simulink model "sampleModel2021"  (R2023a)
settings: Solver=VariableStepAuto  StartTime=0.0  StopTime=10.0  RelTol=1e-3
libraries: hdlsllib x4
settings Model: Creator=user1  LastModifiedBy=user1

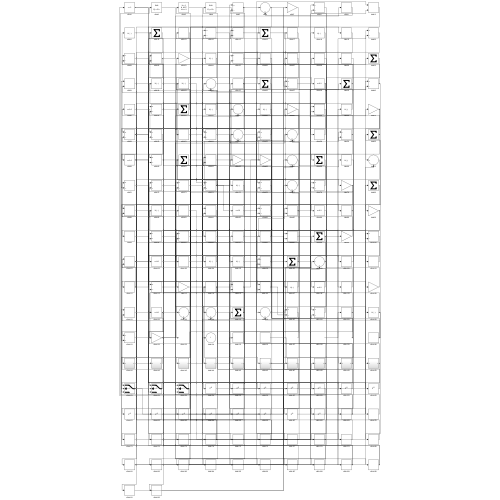
[thumbnail: Simulink's stored preview of the top-level diagram]
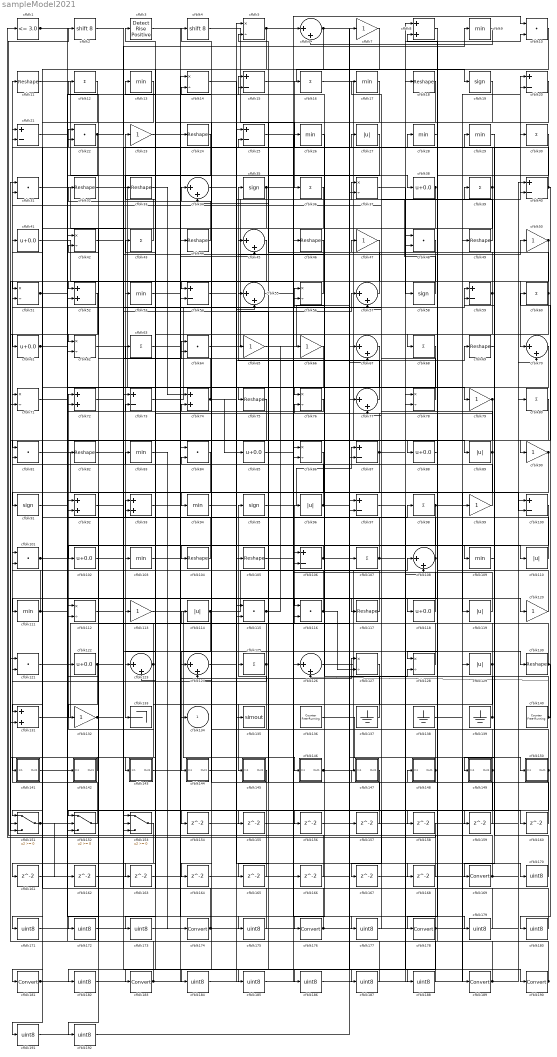
== system sampleModel2021 ==
  cfblk1 : hdlsllib/Logic and Bit Operations/Compare To Constant  relop=<=  const=3.0  OutDataTypeStr=boolean
  cfblk{10,22,31,48,64,81,84,101,115..116,121} (11 alike) : DotProduct  OutDataTypeStr=Inherit: Inherit via internal rule
  cfblk{15,20..21,25,40,54,59,73,87,97,100,106} (12 alike) : Sum  Inputs=+-
  cfblk{38,41,61,85,88,102,118,122} (8 alike) : Bias  Bias=0.0  SaturateOnIntegerOverflow=off
  cfblk{9,13,17,26,28..29,53,83,94,103,109,111} (12 alike) : MinMax
  cfblk{11,18,24,32..33,44,46,49,69,75,82,104..105,117,130} (15 alike) : Reshape
  cfblk{12,16,30,36,39,43,60,63,68,80,98,107,125} (13 alike) : Sum  Inputs=+
  cfblk{6,34,45,55,57,67,70,77,108,123..124,126} (12 alike) : Sum  Inputs=|++
  cfblk{27,89,96,110,114,119,129} (7 alike) : Abs  SaturateOnIntegerOverflow=off
  cfblk{5,14,37,42,51,56,62,71,76,78,86,112,127..128} (14 alike) : Product  Inputs=*/  RndMeth=Zero  SaturateOnIntegerOverflow=on
  cfblk{7,23,47,50,65..66,79,90,99,113,120,132} (12 alike) : Gain
  cfblk{8,52,72,74,92..93,131} (7 alike) : Sum
  cfblk133 : Terminator
  cfblk135 : ToWorkspace  VariableName=simout  SaveFormat=Timeseries  SampleTime=-1
  cfblk136 : hdlsllib/Sources/Counter Free-Running  NumBits=16  tsamp=-1
  cfblk137 : Ground
  cfblk138 : Ground
  cfblk139 : Ground
  cfblk140 : hdlsllib/Sources/Counter Free-Running  NumBits=16  tsamp=-1
  cfblk141 : Subsystem
      settings: LibrarySourceBlock=|
      | hdlsllib/Ports &
      | Subsystems/Subsystem
  cfblk142 : Subsystem
      settings: LibrarySourceBlock=|
      | hdlsllib/Ports &
      | Subsystems/Subsystem
  cfblk143 : Subsystem
      settings: LibrarySourceBlock=|
      | hdlsllib/Ports &
      | Subsystems/Subsystem
  cfblk144 : Subsystem
      settings: LibrarySourceBlock=|
      | hdlsllib/Ports &
      | Subsystems/Subsystem
  cfblk145 : Subsystem
      settings: LibrarySourceBlock=|
      | hdlsllib/Ports &
      | Subsystems/Subsystem
  cfblk146 : Subsystem
      settings: LibrarySourceBlock=|
      | hdlsllib/Ports &
      | Subsystems/Subsystem
  cfblk147 : Subsystem
      settings: LibrarySourceBlock=|
      | hdlsllib/Ports &
      | Subsystems/Subsystem
  cfblk148 : Subsystem
      settings: LibrarySourceBlock=|
      | hdlsllib/Ports &
      | Subsystems/Subsystem
  cfblk149 : Subsystem
      settings: LibrarySourceBlock=|
      | hdlsllib/Ports &
      | Subsystems/Subsystem
  cfblk150 : Subsystem
      settings: LibrarySourceBlock=|
      | hdlsllib/Ports &
      | Subsystems/Subsystem
  cfblk151 : Switch  SaturateOnIntegerOverflow=off  InputSameDT=off
  cfblk152 : Switch  SaturateOnIntegerOverflow=off  InputSameDT=off
  cfblk153 : Switch  SaturateOnIntegerOverflow=off  InputSameDT=off
  cfblk{154..168} (15 alike) : Delay  SampleTime=1
  cfblk{169,174,176,178,181,183,189..190} (8 alike) : DataTypeConversion  SaturateOnIntegerOverflow=off  RndMeth=Floor
  cfblk{170..173,175,177,179..180,182,184..188,191..192} (16 alike) : DataTypeConversion  OutDataTypeStr=uint8  SaturateOnIntegerOverflow=off  RndMeth=Floor
  cfblk{19,35,58,91,95} (5 alike) : Signum
  cfblk2 : ArithShift  BitShiftNumber=8
  cfblk3 : hdlsllib/Logic and Bit Operations/Detect Rise Positive  vinit=0  OutDataTypeStr=boolean
  cfblk4 : ArithShift  BitShiftNumber=8
  cfblk134 : Outport  VectorParamsAs1DForOutWhenUnconnected=off
  wires:
  cfblk73/1 -> cfblk56/1
  cfblk152/1 -> cfblk11/1
  cfblk70/1 -> cfblk104/1
  cfblk11/1 -> cfblk38/1
  cfblk24/1 -> cfblk133/1
  cfblk127/1 -> cfblk72/1
  cfblk77/1 -> cfblk35/1
  cfblk33/1 -> cfblk74/1
  cfblk56/1 -> cfblk51/1
  cfblk150/1(Out1) -> cfblk34/1, cfblk167/1
  cfblk90/1 -> cfblk124/2, cfblk172/1
  cfblk15/1 -> cfblk19/1
  cfblk59/1 -> cfblk94/1, cfblk34/2
  cfblk58/1 -> cfblk20/1
  cfblk26/1 -> cfblk76/1
  cfblk84/1 -> cfblk113/1
  cfblk69/1 -> cfblk149/1(In1)
  cfblk35/1 -> cfblk117/1, cfblk173/1
  cfblk97/1 -> cfblk190/1
  cfblk46/1 -> cfblk52/1
  cfblk16/1 -> cfblk89/1
  cfblk21/1 -> cfblk112/1
  cfblk64/1 -> cfblk37/1
  cfblk116/1 -> cfblk21/1, cfblk127/2
  cfblk121/1 -> cfblk24/1
  cfblk146/1(Out1) -> cfblk108/1, cfblk128/2
  cfblk145/1(Out1) -> cfblk2/1
  cfblk17/1 -> cfblk37/2
  cfblk95/1 -> cfblk87/1
  cfblk138/1 -> cfblk49/1
  cfblk129/1 -> cfblk145/1(In1), cfblk84/2
  cfblk131/1 -> cfblk7/1
  cfblk114/1 -> cfblk144/1(In1), cfblk18/1
  cfblk80/1 -> cfblk181/1
  cfblk19/1 -> cfblk75/1
  cfblk38/1 -> cfblk62/1, cfblk184/1
  cfblk79/1 -> cfblk76/2, cfblk151/3
  cfblk22/1 -> cfblk52/2, cfblk9/1
  cfblk68/1 -> cfblk123/1
  cfblk32/1 -> cfblk107/1
  cfblk43/1 -> cfblk23/1
  cfblk136/1 -> cfblk189/1
  cfblk47/1 -> cfblk176/1
  cfblk89/1 -> cfblk132/1, cfblk31/2
  cfblk130/1 -> cfblk96/1, cfblk180/1
  cfblk148/1(Out1) -> cfblk147/1(In1), cfblk125/1
  cfblk98/1 -> cfblk20/2, cfblk164/1
  cfblk10/1 -> cfblk123/2
  cfblk85/1 -> cfblk46/1
  cfblk109/1 -> cfblk59/1
  cfblk67/1 -> cfblk183/1
  cfblk30/1 -> cfblk118/1
  cfblk76/1 -> cfblk72/2
  cfblk86/1 -> cfblk91/1
  cfblk6/1 -> cfblk131/1, cfblk100/2
  cfblk78/1 -> cfblk51/2
  cfblk41/1 -> cfblk126/1
  cfblk101/1 -> cfblk15/2, cfblk175/1
  cfblk31/1 -> cfblk53/1
  cfblk82/1 -> cfblk50/1
  cfblk106/1 -> cfblk150/1(In1), cfblk102/1
  cfblk122/1 -> cfblk59/2, cfblk152/3
  cfblk126/1 -> cfblk78/1
  cfblk113/1 -> cfblk146/1(In1)
  cfblk99/1 -> cfblk71/1
  cfblk23/1 -> cfblk130/1
  cfblk40/1 -> cfblk16/1, cfblk90/1
  cfblk34/1 -> cfblk30/1
  cfblk71/1 -> cfblk120/1
  cfblk29/1 -> cfblk169/1
  cfblk44/1 -> cfblk32/1
  cfblk149/1(Out1) -> cfblk95/1, cfblk27/1, cfblk182/1
  cfblk110/1 -> cfblk43/1
  cfblk142/1(Out1) -> cfblk141/1(In1)
  cfblk103/1 -> cfblk44/1
  cfblk20/1 -> cfblk54/1
  cfblk1/1 -> cfblk109/1, cfblk79/1
  cfblk45/1 -> cfblk71/2
  cfblk105/1 -> cfblk6/1
  cfblk120/1 -> cfblk21/2
  cfblk91/1 -> cfblk142/1(In1)
  cfblk144/1(Out1) -> cfblk25/1
  cfblk52/1 -> cfblk131/2
  cfblk119/1 -> cfblk106/1
  cfblk137/1 -> cfblk45/1
  cfblk151/1 -> cfblk152/2, cfblk162/1
  cfblk93/1 -> cfblk45/2
  cfblk72/1 -> cfblk153/1
  cfblk4/1 -> cfblk36/1
  cfblk36/1 -> cfblk81/1
  cfblk117/1 -> cfblk33/1
  cfblk8/1 -> cfblk178/1
  cfblk5/1 -> cfblk92/2, cfblk10/1
  cfblk96/1 -> cfblk65/1, cfblk64/2, cfblk168/1
  cfblk60/1 -> cfblk28/1, cfblk143/1(In1)
  cfblk57/1 -> cfblk5/2
  cfblk143/1(Out1) -> cfblk127/1
  cfblk128/1 -> cfblk114/1
  cfblk108/1 -> cfblk13/1, cfblk151/1
  cfblk14/1 -> cfblk55/2
  cfblk66/1 -> cfblk111/1
  cfblk125/1 -> cfblk121/2, cfblk22/1, cfblk93/1
  cfblk100/1 -> cfblk112/2
  cfblk139/1 -> cfblk15/1, cfblk63/1
  cfblk107/1 -> cfblk110/1, cfblk26/1
  cfblk12/1 -> cfblk61/1
  cfblk140/1 -> cfblk56/2, cfblk126/2, cfblk60/1
  cfblk132/1 -> cfblk57/1, cfblk25/2
  cfblk81/1 -> cfblk119/1
  cfblk112/1 -> cfblk98/1
  cfblk74/1 -> cfblk69/1, cfblk22/2, cfblk116/2, cfblk85/1
  cfblk123/1 -> cfblk12/1, cfblk151/2
  cfblk61/1 -> cfblk153/3, cfblk160/1
  cfblk115/1 -> cfblk66/1, cfblk155/1
  cfblk39/1 -> cfblk4/1, cfblk116/1
  cfblk50/1 -> cfblk54/2, cfblk70/1
  cfblk18/1 -> cfblk103/1
  cfblk28/1 -> cfblk68/1
  cfblk51/1 -> cfblk86/2, cfblk115/2
  cfblk37/1 -> cfblk58/1
  cfblk94/1 -> cfblk40/2
  cfblk87/1 -> cfblk3/1, cfblk10/2, cfblk185/1
  cfblk62/1 -> cfblk105/1
  cfblk88/1 -> cfblk128/1
  cfblk13/1 -> cfblk62/2
  cfblk83/1 -> cfblk174/1
  cfblk49/1 -> cfblk17/1
  cfblk102/1 -> cfblk64/1
  cfblk2/1 -> cfblk124/1
  cfblk9/1 -> cfblk6/2
  cfblk65/1 -> cfblk39/1
  cfblk55/1 -> cfblk88/1
  cfblk118/1 -> cfblk77/2
  cfblk104/1 -> cfblk81/2
  cfblk147/1(Out1) -> cfblk152/1
  cfblk111/1 -> cfblk101/1, cfblk93/2
  cfblk141/1(Out1) -> cfblk154/1
  cfblk154/1 -> cfblk86/1
  cfblk155/1 -> cfblk40/1
  cfblk54/1 -> cfblk156/1
  cfblk157/1 -> cfblk55/1
  cfblk3/1 -> cfblk158/1
  cfblk158/1 -> cfblk1/1
  cfblk53/1 -> cfblk159/1
  cfblk159/1 -> cfblk74/2
  cfblk160/1 -> cfblk14/2
  cfblk153/1 -> cfblk161/1
  cfblk161/1 -> cfblk106/2
  cfblk162/1 -> cfblk77/1
  cfblk7/1 -> cfblk163/1
  cfblk163/1 -> cfblk87/2
  cfblk164/1 -> cfblk5/1
  cfblk27/1 -> cfblk165/1
  cfblk165/1 -> cfblk92/1
  cfblk166/1 -> cfblk73/1
  cfblk167/1 -> cfblk70/2
  cfblk168/1 -> cfblk57/2
  cfblk169/1 -> cfblk115/1, cfblk14/1
  cfblk124/1 -> cfblk170/1
  cfblk170/1 -> cfblk29/1
  cfblk48/1 -> cfblk171/1
  cfblk171/1 -> cfblk157/1
  cfblk172/1 -> cfblk48/1
  cfblk173/1 -> cfblk48/2
  cfblk174/1 -> cfblk153/2, cfblk99/1, cfblk82/1
  cfblk175/1 -> cfblk83/1
  cfblk176/1 -> cfblk78/2, cfblk41/1, cfblk100/1, cfblk73/2
  cfblk25/1 -> cfblk177/1
  cfblk177/1 -> cfblk47/1
  cfblk178/1 -> cfblk101/2, cfblk192/1
  cfblk63/1 -> cfblk179/1
  cfblk179/1 -> cfblk8/1
  cfblk180/1 -> cfblk8/2
  cfblk181/1 -> cfblk166/1, cfblk108/2
  cfblk182/1 -> cfblk80/1
  cfblk183/1 -> cfblk134/1, cfblk31/1, cfblk135/1
  cfblk184/1 -> cfblk67/1
  cfblk185/1 -> cfblk67/2
  cfblk42/1 -> cfblk186/1
  cfblk186/1 -> cfblk129/1
  cfblk92/1 -> cfblk187/1
  cfblk187/1 -> cfblk42/1
  cfblk156/1 -> cfblk188/1
  cfblk188/1 -> cfblk42/2
  cfblk189/1 -> cfblk84/1, cfblk122/1
  cfblk190/1 -> cfblk148/1(In1), cfblk121/1
  cfblk75/1 -> cfblk191/1
  cfblk191/1 -> cfblk97/1
  cfblk192/1 -> cfblk97/2

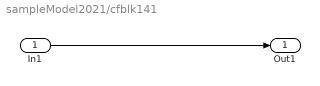
== system sampleModel2021/cfblk141 ==
  In1 : Inport
  Out1 : Outport
  wires:
  In1/1 -> Out1/1

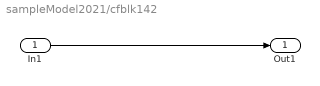
== system sampleModel2021/cfblk142 ==
  In1 : Inport
  Out1 : Outport
  wires:
  In1/1 -> Out1/1

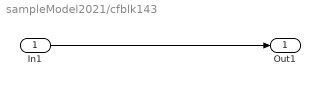
== system sampleModel2021/cfblk143 ==
  In1 : Inport
  Out1 : Outport
  wires:
  In1/1 -> Out1/1

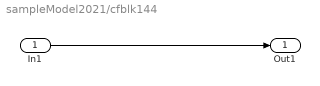
== system sampleModel2021/cfblk144 ==
  In1 : Inport
  Out1 : Outport
  wires:
  In1/1 -> Out1/1

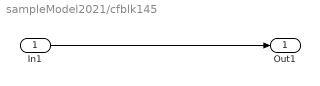
== system sampleModel2021/cfblk145 ==
  In1 : Inport
  Out1 : Outport
  wires:
  In1/1 -> Out1/1

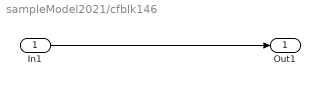
== system sampleModel2021/cfblk146 ==
  In1 : Inport
  Out1 : Outport
  wires:
  In1/1 -> Out1/1

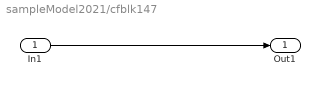
== system sampleModel2021/cfblk147 ==
  In1 : Inport
  Out1 : Outport
  wires:
  In1/1 -> Out1/1

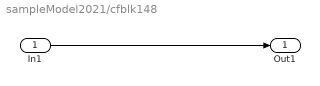
== system sampleModel2021/cfblk148 ==
  In1 : Inport
  Out1 : Outport
  wires:
  In1/1 -> Out1/1

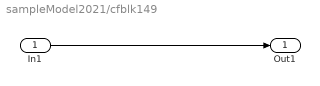
== system sampleModel2021/cfblk149 ==
  In1 : Inport
  Out1 : Outport
  wires:
  In1/1 -> Out1/1

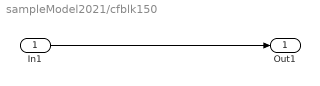
== system sampleModel2021/cfblk150 ==
  In1 : Inport
  Out1 : Outport
  wires:
  In1/1 -> Out1/1
